simulink library "SOEM_EtherCAT_Lib"  (Simulink 8.5)
settings: Solver=ode45  StartTime=0.0  StopTime=10.0  RelTol=1e-3
undefined symbols (not defined in the file): setpoints
settings Model: Creator=RecSet  LastModifiedBy=maxbaeten  CovSaveCumulativeToWorkspaceVar=on  CovSFcnEnable=off

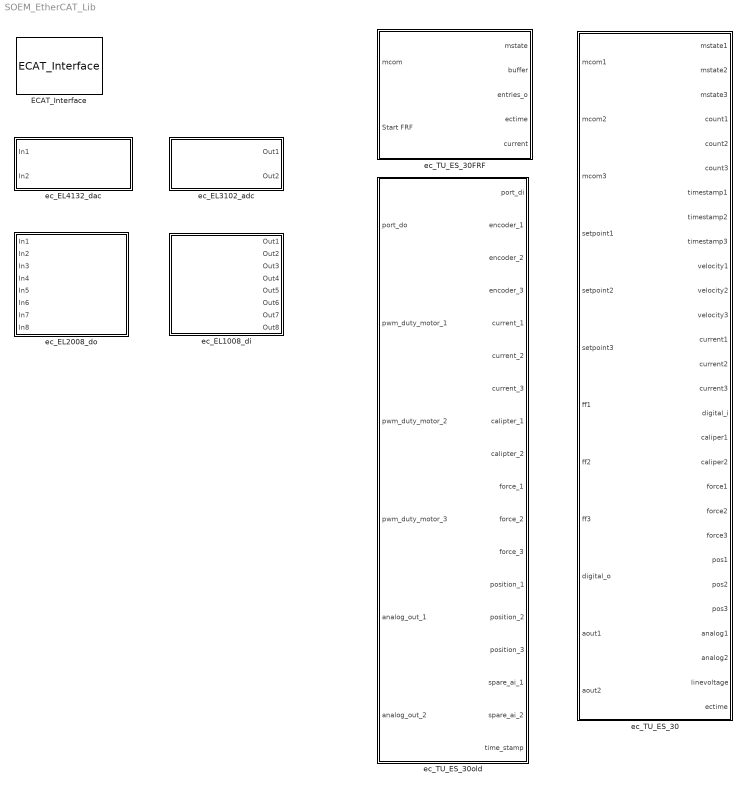
== system SOEM_EtherCAT_Lib ==
  ECAT_Interface : S-Function  Priority=0  StopFcn=|  FunctionName=ECAT_Interface  Parameters=IFINTERFACE,TS  SFunctionDeploymentMode=off  EnableBusSupport=off  mask{IFINTERFACE=eth0, TS=1/1000}
      | t_ = timer('Name','DLL_Unload_timer',...
      |             'ExecutionMode','singleShot',...
      |             'StartDelay',2,...
      |             'StopFcn','try;delete(t_);clear(''t_'');catch;disp(''Unloading DLL Failed!'');end;',...
      |             'TimerFcn','clear mex;'); 
      | start(t_);
      mask prompts: TS "Block sample time [s]"
      mask Callback IFINTERFACE:
      | VAR = get_param(gcb, 'IFINTERFACE');
      | if ~isnan(str2double(VAR))
      |     errordlg('Enter a string!');
      |     set_param(gcb, 'IFINTERFACE', '\Device\NPF_{$KEY}');
      | end
  ec_EL1008_di : Subsystem  mask(EL1008 di){LINKID=1}
      mask prompts: LINKID "Enter link id (>0)"
  ec_EL2008_do : Subsystem  mask(EL2008 do){LINKID=1}
      mask prompts: LINKID "Enter link id (>0)"
  ec_EL3102_adc : Subsystem  mask(EL3102 adc){LINKID=1}
      mask prompts: LINKID "Enter link id (>0)"
  ec_EL4132_dac : Subsystem  mask(EL4132 dac){LINKID=1}
      mask prompts: LINKID "Enter link id (>0)"
  ec_TU_ES_30 : Subsystem  AncestorBlock=SERGIO_Lib/EtherCAT Blocks/ec_TU_ES_30  mask{link_id=1, slave_num=2, resistance=[0.61, 0.61, 0.61], kv=[0.03, 0.03, 0.03], pgain=[2.00, 2.00, 2.00], igain=[2.00, 2.00, 2.00], ilimit=[0.2, 0.2, 0.2], encdir=[1, 1, 1], encres=[1024, 1024, 1024], czero=[2168, 2168, 2168]}
      mask prompts: link_id "Link id (>0)"; slave_num "Slave number (count up from coupler = 1)"; resistance "Motor Resistance"
      mask DialogControl ParameterTabVar0 Prompt: Parameters
  ec_TU_ES_30FRF : Subsystem  AncestorBlock=SERGIO_Lib/EtherCAT Blocks/ec_TU_ES_30FRF  mask{link_id=1, slave_num=2, resistance=[0.61, 0.61, 0.61], kv=[0.03, 0.03, 0.03], pgain=[2.00, 2.00, 2.00], igain=[2.00, 2.00, 2.00], ilimit=[0.2, 0.2, 0.2], encdir=[1, 1, 1], encres=[1024, 1024, 1024], czero=[2168, 2168, 2168], setpts=setpoints, numsets=length(setpoints)}
      mask prompts: link_id "Link id (>0)"; slave_num "Slave number (count up from coupler = 1)"; resistance "Motor Resistance"; setpts "Array of setpoints"; numsets "Number of setpoints"
  ec_TU_ES_30old : Subsystem  AncestorBlock=SERGIO_Lib/EtherCAT Blocks/ec_TU_ES_030old  mask{link_id=1}
      mask prompts: link_id "Link id (>0)"

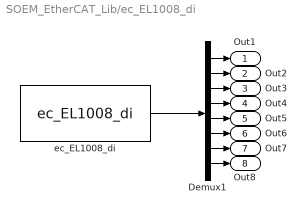
== system SOEM_EtherCAT_Lib/ec_EL1008_di ==
  Demux1 : Demux  Outputs=8
  ec_EL1008_di : S-Function  Priority=1  FunctionName=ec_EL1008_di  Parameters=LINKID  SFunctionDeploymentMode=off  EnableBusSupport=off
  Out1 : Outport
  Out2 : Outport  Port=2
  Out3 : Outport  Port=3
  Out4 : Outport  Port=4
  Out5 : Outport  Port=5
  Out6 : Outport  Port=6
  Out7 : Outport  Port=7
  Out8 : Outport  Port=8
  wires:
  Demux1/3 -> Out3/1
  Demux1/5 -> Out5/1
  Demux1/8 -> Out8/1
  Demux1/2 -> Out2/1
  Demux1/4 -> Out4/1
  Demux1/1 -> Out1/1
  Demux1/6 -> Out6/1
  Demux1/7 -> Out7/1
  ec_EL1008_di/1 -> Demux1/1

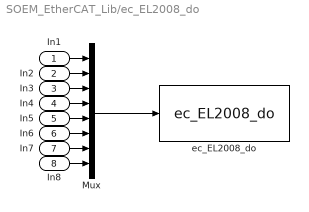
== system SOEM_EtherCAT_Lib/ec_EL2008_do ==
  In1 : Inport
  In2 : Inport  Port=2
  In3 : Inport  Port=3
  In4 : Inport  Port=4
  In5 : Inport  Port=5
  In6 : Inport  Port=6
  In7 : Inport  Port=7
  In8 : Inport  Port=8
  Mux : Mux  Inputs=8
  ec_EL2008_do : S-Function  Priority=1  FunctionName=ec_EL2008_do  Parameters=LINKID  SFunctionDeploymentMode=off  EnableBusSupport=off
  wires:
  In8/1 -> Mux/8
  In6/1 -> Mux/6
  In1/1 -> Mux/1
  In2/1 -> Mux/2
  In7/1 -> Mux/7
  In3/1 -> Mux/3
  In4/1 -> Mux/4
  In5/1 -> Mux/5
  Mux/1 -> ec_EL2008_do/1

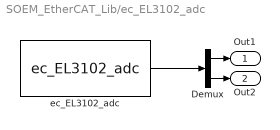
== system SOEM_EtherCAT_Lib/ec_EL3102_adc ==
  Demux : Demux  Outputs=2
  ec_EL3102_adc : S-Function  Priority=1  FunctionName=ec_EL3102_adc  Parameters=LINKID  SFunctionDeploymentMode=off  EnableBusSupport=off
  Out1 : Outport
  Out2 : Outport  Port=2
  wires:
  Demux/1 -> Out1/1
  Demux/2 -> Out2/1
  ec_EL3102_adc/1 -> Demux/1

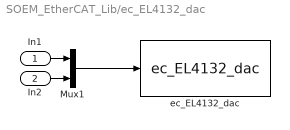
== system SOEM_EtherCAT_Lib/ec_EL4132_dac ==
  In1 : Inport
  In2 : Inport  Port=2
  Mux1 : Mux  Inputs=2
  ec_EL4132_dac : S-Function  Priority=1  FunctionName=ec_EL4132_dac  Parameters=LINKID  SFunctionDeploymentMode=off  EnableBusSupport=off
  wires:
  Mux1/1 -> ec_EL4132_dac/1
  In2/1 -> Mux1/2
  In1/1 -> Mux1/1

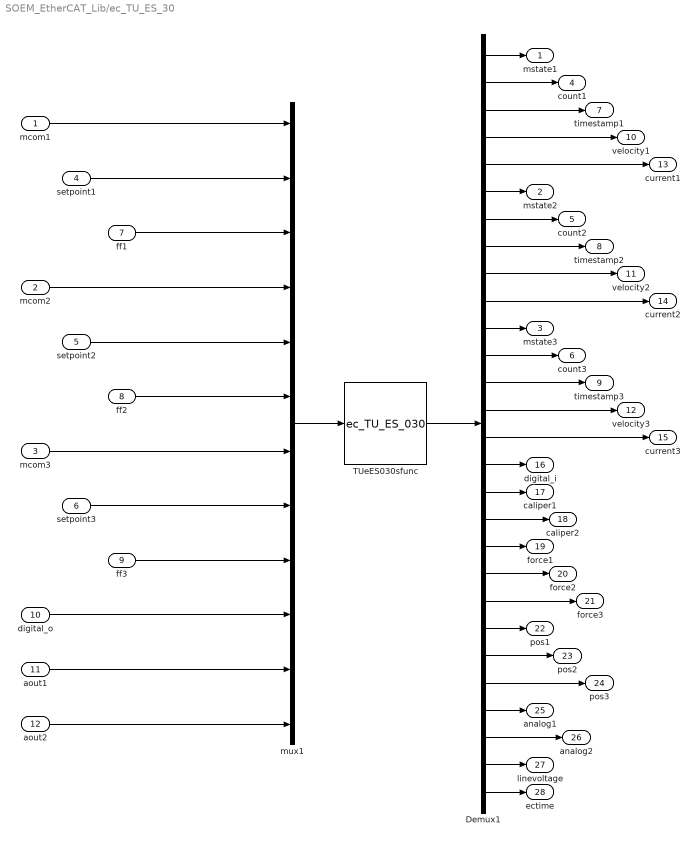
== system SOEM_EtherCAT_Lib/ec_TU_ES_30 ==
  mcom1 : Inport
  mcom2 : Inport  Port=2
  mcom3 : Inport  Port=3
  setpoint1 : Inport  Port=4
  setpoint2 : Inport  Port=5
  setpoint3 : Inport  Port=6
  ff1 : Inport  Port=7
  ff2 : Inport  Port=8
  ff3 : Inport  Port=9
  digital_o : Inport  Port=10
  aout1 : Inport  Port=11
  aout2 : Inport  Port=12
  Demux1 : Demux  Outputs=28
  TUeES030sfunc : S-Function  FunctionName=ec_TU_ES_030  Parameters=link_id, slave_num, resistance, kv,pgain,igain,ilimit,encdir,encres,czero  SFunctionDeploymentMode=off  EnableBusSupport=off  mask{link_id=link_id, slave_num=slave_num, resistance=resistance, kv=kv, pgain=pgain, igain=igain, ilimit=ilimit, encdir=encdir, encres=encres, czero=czero}
      mask prompts: link_id "Link id (start from 1)"; slave_num "Slave number (count up from coupler = 1)"
  mux1 : Mux  Inputs=12
  mstate1 : Outport
  mstate2 : Outport  Port=2
  mstate3 : Outport  Port=3
  count1 : Outport  Port=4
  count2 : Outport  Port=5
  count3 : Outport  Port=6
  timestamp1 : Outport  Port=7
  timestamp2 : Outport  Port=8
  timestamp3 : Outport  Port=9
  velocity1 : Outport  Port=10
  velocity2 : Outport  Port=11
  velocity3 : Outport  Port=12
  current1 : Outport  Port=13
  current2 : Outport  Port=14
  current3 : Outport  Port=15
  digital_i : Outport  Port=16
  caliper1 : Outport  Port=17
  caliper2 : Outport  Port=18
  force1 : Outport  Port=19
  force2 : Outport  Port=20
  force3 : Outport  Port=21
  pos1 : Outport  Port=22
  pos2 : Outport  Port=23
  pos3 : Outport  Port=24
  analog1 : Outport  Port=25
  analog2 : Outport  Port=26
  linevoltage : Outport  Port=27
  ectime : Outport  Port=28
  wires:
  Demux1/28 -> ectime/1
  Demux1/27 -> linevoltage/1
  Demux1/26 -> analog2/1
  Demux1/25 -> analog1/1
  Demux1/24 -> pos3/1
  Demux1/23 -> pos2/1
  Demux1/22 -> pos1/1
  Demux1/21 -> force3/1
  Demux1/20 -> force2/1
  Demux1/19 -> force1/1
  Demux1/18 -> caliper2/1
  Demux1/17 -> caliper1/1
  Demux1/16 -> digital_i/1
  Demux1/15 -> current3/1
  Demux1/14 -> velocity3/1
  Demux1/13 -> timestamp3/1
  Demux1/12 -> count3/1
  Demux1/11 -> mstate3/1
  Demux1/10 -> current2/1
  Demux1/9 -> velocity2/1
  Demux1/8 -> timestamp2/1
  Demux1/7 -> count2/1
  Demux1/6 -> mstate2/1
  Demux1/5 -> current1/1
  Demux1/4 -> velocity1/1
  Demux1/3 -> timestamp1/1
  Demux1/2 -> count1/1
  Demux1/1 -> mstate1/1
  TUeES030sfunc/1 -> Demux1/1
  aout2/1 -> mux1/12
  aout1/1 -> mux1/11
  digital_o/1 -> mux1/10
  ff3/1 -> mux1/9
  setpoint3/1 -> mux1/8
  mcom3/1 -> mux1/7
  ff2/1 -> mux1/6
  setpoint2/1 -> mux1/5
  mcom2/1 -> mux1/4
  ff1/1 -> mux1/3
  setpoint1/1 -> mux1/2
  mcom1/1 -> mux1/1
  mux1/1 -> TUeES030sfunc/1

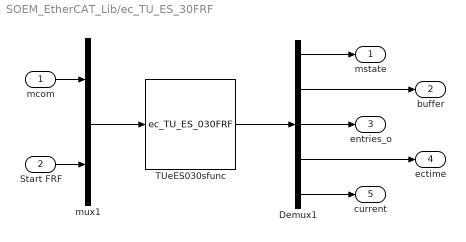
== system SOEM_EtherCAT_Lib/ec_TU_ES_30FRF ==
  mcom : Inport
  Start FRF : Inport  Port=2
  Demux1 : Demux  Outputs=[1 1 1 1 22]
  TUeES030sfunc : S-Function  FunctionName=ec_TU_ES_030FRF  Parameters=link_id, slave_num, resistance, kv,pgain,igain,ilimit,encdir,encres,czero, setpts,numsets  SFunctionDeploymentMode=off  EnableBusSupport=off  mask{link_id=link_id, slave_num=slave_num, resistance=resistance, kv=kv, pgain=pgain, igain=igain, ilimit=ilimit, encdir=encdir, encres=encres, czero=czero, setpts=setpts, numsets=numsets}
      mask prompts: link_id "Link id (start from 1)"; slave_num "Slave number (count from coupler = 1)"; setpts "Array of setpoints"; numsets "Number of setpoints"
  mux1 : Mux  Inputs=2
  mstate : Outport
  buffer : Outport  Port=2
  entries_o : Outport  Port=3
  ectime : Outport  Port=4
  current : Outport  Port=5
  wires:
  Demux1/5 -> current/1
  Demux1/4 -> ectime/1
  Demux1/3 -> entries_o/1
  Demux1/2 -> buffer/1
  Demux1/1 -> mstate/1
  TUeES030sfunc/1 -> Demux1/1
  Start FRF/1 -> mux1/2
  mcom/1 -> mux1/1
  mux1/1 -> TUeES030sfunc/1

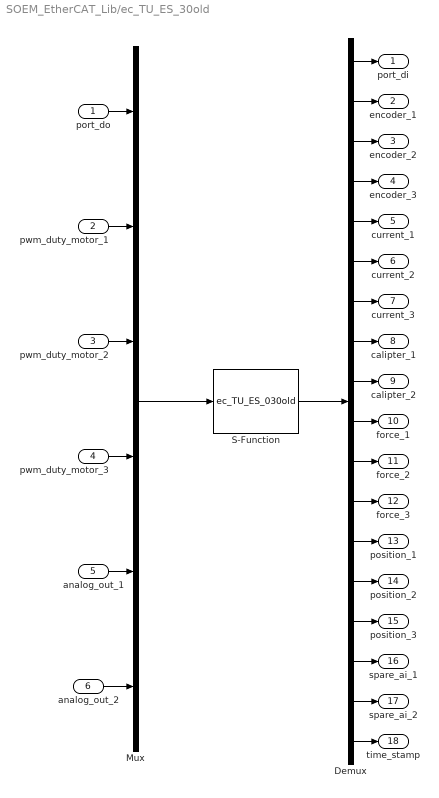
== system SOEM_EtherCAT_Lib/ec_TU_ES_30old ==
  port_do : Inport
  pwm_duty_motor_1 : Inport  Port=2
  pwm_duty_motor_2 : Inport  Port=3
  pwm_duty_motor_3 : Inport  Port=4
  analog_out_1 : Inport  Port=5
  analog_out_2 : Inport  Port=6
  Demux : Demux  Outputs=18
  Mux : Mux  Inputs=6
  S-Function : S-Function  FunctionName=ec_TU_ES_030old  Parameters=link_id  SFunctionDeploymentMode=off  EnableBusSupport=off  mask{link_id=link_id}
      mask prompts: link_id "Link id (start from 1)"
  port_di : Outport
  encoder_1 : Outport  Port=2
  encoder_2 : Outport  Port=3
  encoder_3 : Outport  Port=4
  current_1 : Outport  Port=5
  current_2 : Outport  Port=6
  current_3 : Outport  Port=7
  calipter_1 : Outport  Port=8
  calipter_2 : Outport  Port=9
  force_1 : Outport  Port=10
  force_2 : Outport  Port=11
  force_3 : Outport  Port=12
  position_1 : Outport  Port=13
  position_2 : Outport  Port=14
  position_3 : Outport  Port=15
  spare_ai_1 : Outport  Port=16
  spare_ai_2 : Outport  Port=17
  time_stamp : Outport  Port=18
  wires:
  Mux/1 -> S-Function/1
  S-Function/1 -> Demux/1
  port_do/1 -> Mux/1
  pwm_duty_motor_1/1 -> Mux/2
  Demux/1 -> port_di/1
  pwm_duty_motor_2/1 -> Mux/3
  pwm_duty_motor_3/1 -> Mux/4
  analog_out_1/1 -> Mux/5
  analog_out_2/1 -> Mux/6
  Demux/2 -> encoder_1/1
  Demux/3 -> encoder_2/1
  Demux/4 -> encoder_3/1
  Demux/5 -> current_1/1
  Demux/6 -> current_2/1
  Demux/7 -> current_3/1
  Demux/8 -> calipter_1/1
  Demux/9 -> calipter_2/1
  Demux/10 -> force_1/1
  Demux/11 -> force_2/1
  Demux/12 -> force_3/1
  Demux/13 -> position_1/1
  Demux/14 -> position_2/1
  Demux/15 -> position_3/1
  Demux/16 -> spare_ai_1/1
  Demux/17 -> spare_ai_2/1
  Demux/18 -> time_stamp/1
